simulink model "env_extQ16"  (R2022b)
settings: Solver=VariableStepAuto  StartTime=0.0  StopTime=30  RelTol=1e-3
values from neighbouring files (symbols this model uses):
  B = 8    [variables.m]    (also in variables16.m)
  cordic_delay = 20    [variables.m]    (also in variables16.m)
  e_val = 1/l2    [variables.m]    (also in variables16.m)
  exp_fract_len_homo = 26    [variables.m]    (also in variables16.m = 10)
  exp_word_len_homo = 32    [variables.m]    (also in variables16.m = 16)
  explarge_delay = 3    [variables.m]    (also in variables16.m)
  fft_len_hilb = 2048    [variables.m]    (also in variables16.m)
  fft_length = 4096    [variables.m]    (also in variables16.m)
  frac_bit_l2 = 30    [variables.m]    (also in variables16.m = 14)
  frac_bit_l3 = 29    [variables.m]    (also in variables16.m = 13)
  frac_bit_l4 = 28    [variables.m]    (also in variables16.m = 12)
  grp_delay_hilb = 11    [variables.m]    (also in variables16.m)
  grp_delay_homo = 13    [variables.m]    (also in variables16.m)
  grp_delay_psd = 19    [variables.m]    (also in variables16.m)
  grp_delay_swt = 12    [variables.m]    (also in variables16.m)
  l2 = log(2)    [variables.m]    (also in variables16.m)
  l2e = 1/log2(exp(1))    [variables.m]    (also in variables16.m)
  log2_table = log2((2^(B-1) : 2^(B)) / 2^(B - 1))    [variables.m]    (also in variables16.m)
  log_fract_len_homo = 31    [variables.m]    (also in variables16.m = 15)
  log_latency = 21    [variables.m]    (also in variables16.m)
  log_word_len = 48    [variables.m]    (also in variables16.m = 24)
  log_word_len_homo = 32    [variables.m]    (also in variables16.m = 16)
  NLZLUT = B-ceil(log2((1:2^B)))    [variables.m]    (also in variables16.m)
  scale = 1.0 / (fs * sum(window_val.*window_val))    [variables.m]    (also in variables16.m)
  win_dim = 64    [variables.m]    (also in variables16.m)
  window_dim = 100    [variables.m]    (also in variables16.m)
undefined symbols (not defined in the file or in its folder): C, c, fl_high_index, fl_low_index, HiD, hilbert_fifo_full, LoD, psd_fifo_full, SFVC784, swt_fifo_full, XCK26, xlfda_numerator
libraries: hdlBasic x626, hdlDSPIP x12, hdlUtilities x2, dspsnks4 x1, dspvision x1, vmcUtilities x1
(part 7 of 7)

== system env_extQ16/env_extr/SWT/shannonE/log2/normalize_input/stage7 ==
  v_in : Inport
  n_shift_in : Inport  Port=2
  mem_data_in : Inport  Port=3
  en : Inport  Port=4
  AddSub1 : hdlBasic/AddSub  mode=Addition  use_carryin=off  use_carryout=off  en=on  latency=1  precision=Full  arith_type=Unsigned  n_bits=16  bin_pt=14  quantization=Truncate  overflow=Wrap  use_behavioral_HDL=off  hw_selection=Fabric  pipelined=off  XmcBlockStatus=1  maskContainerNames=tabcontainer1  block_type=addsub  block_config=sysgen:Addsub_config
  Delay2 : hdlBasic/Delay  rst=off  en=on  latency=1  reg_retiming=off  XmcBlockStatus=1  maskContainerNames=group1  block_type=delay  block_config=sysgen:Delay_config
  Mux : hdlBasic/Mux  inputs=9  en=on  latency=1  precision=Full  arith_type=Unsigned  n_bits=16  bin_pt=14  quantization=Truncate  overflow=Wrap  XmcBlockStatus=1  maskContainerNames=tabcontainer1  block_type=mux  block_config=sysgen:Mux_config
  Shift1 : hdlBasic/Shift  shift_dir=Left  shift_bits=8  en=on  latency=1  precision=Full  arith_type="Signed  (2's comp)"  n_bits=16  bin_pt=14  quantization=Truncate  overflow=Wrap  XmcBlockStatus=1  maskContainerNames=group2  block_type=shift  block_config=sysgen:Shift_config
  Shift2 : hdlBasic/Shift  shift_dir=Left  shift_bits=1  en=on  latency=1  precision=Full  arith_type="Signed  (2's comp)"  n_bits=16  bin_pt=14  quantization=Truncate  overflow=Wrap  XmcBlockStatus=1  maskContainerNames=group2  block_type=shift  block_config=sysgen:Shift_config
  Shift3 : hdlBasic/Shift  shift_dir=Left  shift_bits=2  en=on  latency=1  precision=Full  arith_type="Signed  (2's comp)"  n_bits=16  bin_pt=14  quantization=Truncate  overflow=Wrap  XmcBlockStatus=1  maskContainerNames=group2  block_type=shift  block_config=sysgen:Shift_config
  Shift4 : hdlBasic/Shift  shift_dir=Left  shift_bits=3  en=on  latency=1  precision=Full  arith_type="Signed  (2's comp)"  n_bits=16  bin_pt=14  quantization=Truncate  overflow=Wrap  XmcBlockStatus=1  maskContainerNames=group2  block_type=shift  block_config=sysgen:Shift_config
  Shift5 : hdlBasic/Shift  shift_dir=Left  shift_bits=4  en=on  latency=1  precision=Full  arith_type="Signed  (2's comp)"  n_bits=16  bin_pt=14  quantization=Truncate  overflow=Wrap  XmcBlockStatus=1  maskContainerNames=group2  block_type=shift  block_config=sysgen:Shift_config
  Shift6 : hdlBasic/Shift  shift_dir=Left  shift_bits=5  en=on  latency=1  precision=Full  arith_type="Signed  (2's comp)"  n_bits=16  bin_pt=14  quantization=Truncate  overflow=Wrap  XmcBlockStatus=1  maskContainerNames=group2  block_type=shift  block_config=sysgen:Shift_config
  Shift7 : hdlBasic/Shift  shift_dir=Left  shift_bits=6  en=on  latency=1  precision=Full  arith_type="Signed  (2's comp)"  n_bits=16  bin_pt=14  quantization=Truncate  overflow=Wrap  XmcBlockStatus=1  maskContainerNames=group2  block_type=shift  block_config=sysgen:Shift_config
  Shift8 : hdlBasic/Shift  shift_dir=Left  shift_bits=7  en=on  latency=1  precision=Full  arith_type="Signed  (2's comp)"  n_bits=16  bin_pt=14  quantization=Truncate  overflow=Wrap  XmcBlockStatus=1  maskContainerNames=group2  block_type=shift  block_config=sysgen:Shift_config
  Shift9 : hdlBasic/Shift  shift_dir=Left  shift_bits=0  en=on  latency=1  precision=Full  arith_type="Signed  (2's comp)"  n_bits=16  bin_pt=14  quantization=Truncate  overflow=Wrap  XmcBlockStatus=1  maskContainerNames=group2  block_type=shift  block_config=sysgen:Shift_config
  Slice1 : hdlBasic/Slice  nbits=B  boolean_output=off  mode=Upper Bit Location + Width  bit1=0  base1=MSB of Input  bit0=8  base0=LSB of Input  XmcBlockStatus=1  maskContainerNames=group1  block_type=slice  block_config=sysgen:Slice_config
  v_out : Outport
  n_shift_out : Outport  Port=2
  mem_addr : Outport  Port=3
  wires:
  Shift7/1 -> Mux/8
  Shift4/1 -> Mux/5
  v_in/1 -> Slice1/1, Shift1/1, Shift8/1, Shift7/1, Shift6/1, Shift5/1, Shift4/1, Shift3/1, Shift2/1, Shift9/1
  Shift6/1 -> Mux/7
  Shift2/1 -> Mux/3
  Shift8/1 -> Mux/9
  Shift3/1 -> Mux/4
  Shift5/1 -> Mux/6
  Slice1/1 -> mem_addr/1
  Shift1/1 -> Mux/10
  Mux/1 -> v_out/1
  AddSub1/1 -> n_shift_out/1
  n_shift_in/1 -> Delay2/1
  mem_data_in/1 -> AddSub1/2, Mux/1
  Delay2/1 -> AddSub1/1
  Shift9/1 -> Mux/2
  en/1 -> Shift8/2, Shift7/2, Shift6/2, Shift5/2, Shift4/2, Shift2/2, Mux/11, AddSub1/3, Delay2/2, Shift9/2, Shift3/2, Shift1/2

== system env_extQ16/env_extr/SWT/shannonE/log2/normalize_input/stage8 ==
  v_in : Inport
  n_shift_in : Inport  Port=2
  mem_data_in : Inport  Port=3
  en : Inport  Port=4
  AddSub1 : hdlBasic/AddSub  mode=Subtraction  use_carryin=off  use_carryout=off  en=on  latency=1  precision=Full  arith_type=Unsigned  n_bits=16  bin_pt=14  quantization=Truncate  overflow=Wrap  use_behavioral_HDL=off  hw_selection=Fabric  pipelined=off  XmcBlockStatus=1  maskContainerNames=tabcontainer1  block_type=addsub  block_config=sysgen:Addsub_config
  AddSub2 : hdlBasic/AddSub  mode=Subtraction  use_carryin=off  use_carryout=off  en=on  latency=1  precision=Full  arith_type=Unsigned  n_bits=16  bin_pt=14  quantization=Truncate  overflow=Wrap  use_behavioral_HDL=off  hw_selection=Fabric  pipelined=off  XmcBlockStatus=1  maskContainerNames=tabcontainer1  block_type=addsub  block_config=sysgen:Addsub_config
  Constant1 : hdlBasic/Constant  const=log_word_len-log_fract_len-1  gui_display_data_type=Fixed-point  arith_type=Unsigned  n_bits=4  bin_pt=0  preci_type=Single  exp_width=8  frac_width=24  explicit_period=off  period=1  XmcBlockStatus=1  maskContainerNames=tabcontainer1  block_type=constant  block_config=sysgen:Constant_config
  Mux : hdlBasic/Mux  inputs=9  en=on  latency=1  precision=Full  arith_type=Unsigned  n_bits=16  bin_pt=14  quantization=Truncate  overflow=Wrap  XmcBlockStatus=1  maskContainerNames=tabcontainer1  block_type=mux  block_config=sysgen:Mux_config
  Reinterpret : hdlBasic/Reinterpret  force_arith_type=off  arith_type=Unsigned  force_bin_pt=on  bin_pt=log_word_len-1  XmcBlockStatus=1  maskContainerNames=group1  block_type=reinterpret  block_config=sysgen:Reinterpret_config
  Shift1 : hdlBasic/Shift  shift_dir=Left  shift_bits=8  en=on  latency=1  precision=Full  arith_type="Signed  (2's comp)"  n_bits=16  bin_pt=14  quantization=Truncate  overflow=Wrap  XmcBlockStatus=1  maskContainerNames=group2  block_type=shift  block_config=sysgen:Shift_config
  Shift2 : hdlBasic/Shift  shift_dir=Left  shift_bits=1  en=on  latency=1  precision=Full  arith_type="Signed  (2's comp)"  n_bits=16  bin_pt=14  quantization=Truncate  overflow=Wrap  XmcBlockStatus=1  maskContainerNames=group2  block_type=shift  block_config=sysgen:Shift_config
  Shift3 : hdlBasic/Shift  shift_dir=Left  shift_bits=2  en=on  latency=1  precision=Full  arith_type="Signed  (2's comp)"  n_bits=16  bin_pt=14  quantization=Truncate  overflow=Wrap  XmcBlockStatus=1  maskContainerNames=group2  block_type=shift  block_config=sysgen:Shift_config
  Shift4 : hdlBasic/Shift  shift_dir=Left  shift_bits=3  en=on  latency=1  precision=Full  arith_type="Signed  (2's comp)"  n_bits=16  bin_pt=14  quantization=Truncate  overflow=Wrap  XmcBlockStatus=1  maskContainerNames=group2  block_type=shift  block_config=sysgen:Shift_config
  Shift5 : hdlBasic/Shift  shift_dir=Left  shift_bits=4  en=on  latency=1  precision=Full  arith_type="Signed  (2's comp)"  n_bits=16  bin_pt=14  quantization=Truncate  overflow=Wrap  XmcBlockStatus=1  maskContainerNames=group2  block_type=shift  block_config=sysgen:Shift_config
  Shift6 : hdlBasic/Shift  shift_dir=Left  shift_bits=5  en=on  latency=1  precision=Full  arith_type="Signed  (2's comp)"  n_bits=16  bin_pt=14  quantization=Truncate  overflow=Wrap  XmcBlockStatus=1  maskContainerNames=group2  block_type=shift  block_config=sysgen:Shift_config
  Shift7 : hdlBasic/Shift  shift_dir=Left  shift_bits=6  en=on  latency=1  precision=Full  arith_type="Signed  (2's comp)"  n_bits=16  bin_pt=14  quantization=Truncate  overflow=Wrap  XmcBlockStatus=1  maskContainerNames=group2  block_type=shift  block_config=sysgen:Shift_config
  Shift8 : hdlBasic/Shift  shift_dir=Left  shift_bits=7  en=on  latency=1  precision=Full  arith_type="Signed  (2's comp)"  n_bits=16  bin_pt=14  quantization=Truncate  overflow=Wrap  XmcBlockStatus=1  maskContainerNames=group2  block_type=shift  block_config=sysgen:Shift_config
  Shift9 : hdlBasic/Shift  shift_dir=Left  shift_bits=0  en=on  latency=1  precision=Full  arith_type="Signed  (2's comp)"  n_bits=16  bin_pt=14  quantization=Truncate  overflow=Wrap  XmcBlockStatus=1  maskContainerNames=group2  block_type=shift  block_config=sysgen:Shift_config
  Slice1 : hdlBasic/Slice  nbits=B  boolean_output=off  mode=Upper Bit Location + Width  bit1=0  base1=MSB of Input  bit0=8  base0=LSB of Input  XmcBlockStatus=1  maskContainerNames=group1  block_type=slice  block_config=sysgen:Slice_config
  v_out : Outport
  n_shift_out : Outport  Port=2
  mem_addr : Outport  Port=3
  wires:
  Shift7/1 -> Mux/8
  Shift4/1 -> Mux/5
  Shift6/1 -> Mux/7
  Shift2/1 -> Mux/3
  Shift8/1 -> Mux/9
  Shift3/1 -> Mux/4
  Shift5/1 -> Mux/6
  Mux/1 -> Reinterpret/1
  n_shift_in/1 -> AddSub2/2
  AddSub2/1 -> AddSub1/1
  Constant1/1 -> AddSub2/1
  mem_data_in/1 -> Mux/1, AddSub1/2
  v_in/1 -> Slice1/1, Shift1/1, Shift8/1, Shift7/1, Shift6/1, Shift5/1, Shift4/1, Shift3/1, Shift2/1, Shift9/1
  Slice1/1 -> mem_addr/1
  Reinterpret/1 -> v_out/1
  Shift1/1 -> Mux/10
  AddSub1/1 -> n_shift_out/1
  Shift9/1 -> Mux/2
  en/1 -> Shift8/2, Shift6/2, Shift5/2, Shift4/2, Shift3/2, Shift2/2, Mux/11, AddSub1/3, AddSub2/3, Shift9/2, Shift7/2, Shift1/2
